simulink model "testMPCWalkingPatternGen"  (R2019b)
settings: Solver=VariableStepAuto  StartTime=0.0  StopTime=10.0  RelTol=1e-3
undefined symbols (not defined in the file or in its folder): numOutputs, predictionHorizon, stepLength, stepTime, stepWidth, Ts, zc
libraries: cstblocks x2, mpclib x2, simulink x1
settings Model: Creator=csantacr  LastModifiedBy=scastro
settings DataIOCC: ReturnWorkspaceOutputs=off
settings DebuggingCC: ArithmeticOperatorsInVariantConditions=warning
settings SFSimCC: CustomCodeUndefinedFunction=UseInterfaceOnly

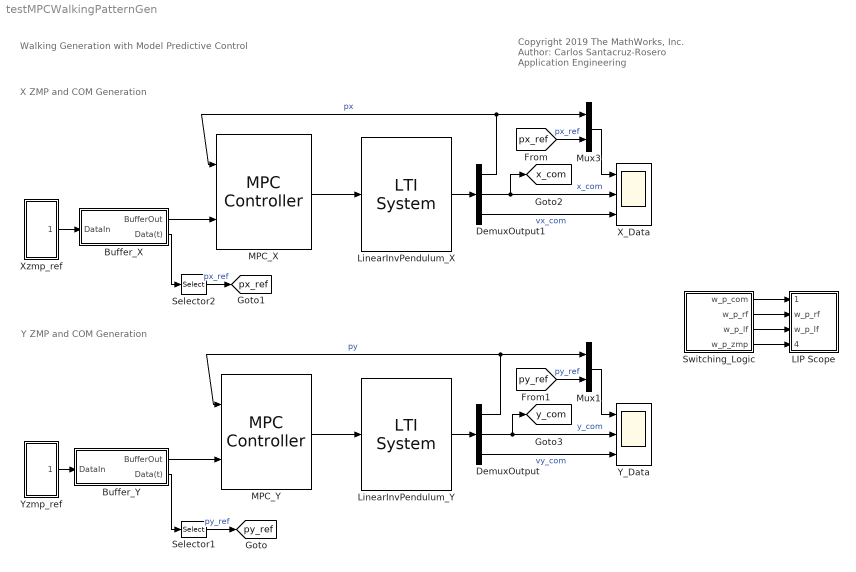
== system testMPCWalkingPatternGen ==
  note: Copyright 2019 The MathWorks, Inc.
      | Author: Carlos Santacruz-Rosero
      | Application Engineering
  note: Walking Generation with Model Predictive Control
  note: Y ZMP and COM Generation
  note: X ZMP and COM Generation
  Buffer_X : Subsystem
  Buffer_Y : Subsystem
  DemuxOutput : Demux  Outputs=3
  DemuxOutput1 : Demux  Outputs=3
  LIP Scope : Subsystem
  LinearInvPendulum_X : cstblocks/LTI System  sys=lip_x_d  IC=[0;0;0]  mask(LTI Block){}
      mask Display:
      | % This is a new mask on top of the base mask.
      | % Use "View base mask" link below to see the base mask.
      | image('lipm.jpg')
  LinearInvPendulum_Y : cstblocks/LTI System  sys=lip_y_d  IC=[0;0;0]  mask(LTI Block){}
      mask Display:
      | % This is a new mask on top of the base mask.
      | % Use "View base mask" link below to see the base mask.
      | image('lipm.jpg');
  MPC_X : mpclib/MPC Controller  SCDEnableBlockLinearizationSpecification=on  mpcobj=mpc1  is_multiple=0  enable_value=0  return_u0=off  updateMPCinCallerWorkspace=on  md_inport=off  mv_inport=off  uref_inport=off  return_cost=off  return_mvseq=off  return_qpstatus=off  return_xseq=off  return_state=off  return_ovseq=off  state_inport=off  umin_inport=off  umax_inport=off  ymin_inport=off  ymax_inport=off  cc_inport=off  ywt_inport=off  uwt_inport=off  duwt_inport=off  rhoeps_inport=off  pm_inport=off  MaximumP=10  HorizonChoice=FixedHorizon  n_ts=0.005  n_p=300  n_mv=1  n_md=0  n_ud=0  n_mo=1  n_uo=2  BlockDataType=double  SampleTimeInherited=off  switch_inport=off
  MPC_Y : mpclib/MPC Controller  SCDEnableBlockLinearizationSpecification=on  mpcobj=mpc1  is_multiple=0  enable_value=0  return_u0=off  updateMPCinCallerWorkspace=on  md_inport=off  mv_inport=off  uref_inport=off  return_cost=off  return_mvseq=off  return_qpstatus=off  return_xseq=off  return_state=off  return_ovseq=off  state_inport=off  umin_inport=off  umax_inport=off  ymin_inport=off  ymax_inport=off  cc_inport=off  ywt_inport=off  uwt_inport=off  duwt_inport=off  rhoeps_inport=off  pm_inport=off  MaximumP=10  HorizonChoice=FixedHorizon  n_ts=0.005  n_p=300  n_mv=1  n_md=0  n_ud=0  n_mo=1  n_uo=2  BlockDataType=double  SampleTimeInherited=off  switch_inport=off
  Mux1 : Mux  Inputs=2
  Mux3 : Mux  Inputs=2
  Selector1 : Selector  InputPortWidth=3  IndexOptions=Index vector (dialog)  Indices=[1]  OutputSizes=1
  Selector2 : Selector  InputPortWidth=3  IndexOptions=Index vector (dialog)  Indices=[1]  OutputSizes=1
  Switching_Logic : Subsystem
  X_Data : Scope  NumInputPorts=3
  Xzmp_ref : Subsystem
  Y_Data : Scope  NumInputPorts=3
  Yzmp_ref : Subsystem
  tag scope: px_ref=global, py_ref=global, x_com=global, y_com=global
  wires:
  LinearInvPendulum_Y/1 -> DemuxOutput/1
  DemuxOutput/1 -> Mux1/1, MPC_Y/1  "py"
  DemuxOutput/2 -> Y_Data/2, [y_com]  "y_com"
  DemuxOutput/3 -> Y_Data/3  "vy_com"
  MPC_Y/1 -> LinearInvPendulum_Y/1
  [py_ref] -> Mux1/2  "py_ref"
  Mux1/1 -> Y_Data/1
  Buffer_Y/2(Data(t)) -> Selector1/1
  Buffer_Y/1(BufferOut) -> MPC_Y/2
  Buffer_X/1(BufferOut) -> MPC_X/2
  Buffer_X/2(Data(t)) -> Selector2/1
  MPC_X/1 -> LinearInvPendulum_X/1
  Mux3/1 -> X_Data/1
  [px_ref] -> Mux3/2  "px_ref"
  DemuxOutput1/3 -> X_Data/3  "vx_com"
  DemuxOutput1/2 -> X_Data/2, [x_com]  "x_com"
  DemuxOutput1/1 -> Mux3/1, MPC_X/1  "px"
  LinearInvPendulum_X/1 -> DemuxOutput1/1
  Xzmp_ref/1(X_ref) -> Buffer_X/1(DataIn)
  Yzmp_ref/1(Y_ref) -> Buffer_Y/1(DataIn)
  Selector2/1 -> [px_ref]  "px_ref"
  Selector1/1 -> [py_ref]  "py_ref"
  Switching_Logic/1(w_p_com) -> LIP Scope/1(w_p_com)
  Switching_Logic/2(w_p_rf) -> LIP Scope/2(w_p_rf)
  Switching_Logic/3(w_p_lf) -> LIP Scope/3(w_p_lf)
  Switching_Logic/4(w_p_zmp) -> LIP Scope/4(w_p_zmp)

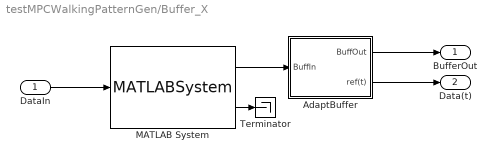
== system testMPCWalkingPatternGen/Buffer_X ==
  DataIn : Inport
  AdaptBuffer : Subsystem
  MATLAB System : MATLABSystem  System=FIFOBuffer  Capacity=predictionHorizon  NumStates=numOutputs  SampleTime=Ts  FillBufferAtStartup=on  BufferStartupFillupData=zeros(numOutputs,predictionHorizon)  SimulateUsing=Code generation
      mask Type: FIFOBuffer
      mask Display:
      | disp('FIFOBuffer');
      | port_label('input',1,'dataIn');
      | port_label('output',1,'buffer');
      | port_label('output',2,'isFull');
  Terminator : Terminator
  BufferOut : Outport
  Data(t) : Outport  Port=2
  wires:
  AdaptBuffer/2(ref(t)) -> Data(t)/1
  DataIn/1 -> MATLAB System/1
  MATLAB System/2 -> Terminator/1
  AdaptBuffer/1(BuffOut) -> BufferOut/1
  MATLAB System/1 -> AdaptBuffer/1(BuffIn)

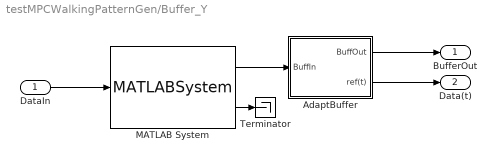
== system testMPCWalkingPatternGen/Buffer_Y ==
  DataIn : Inport
  AdaptBuffer : Subsystem
  MATLAB System : MATLABSystem  System=FIFOBuffer  Capacity=predictionHorizon  NumStates=numOutputs  SampleTime=Ts  FillBufferAtStartup=on  BufferStartupFillupData=zeros(numOutputs,predictionHorizon)  SimulateUsing=Code generation
      mask Type: FIFOBuffer
      mask Display:
      | disp('FIFOBuffer');
      | port_label('input',1,'dataIn');
      | port_label('output',1,'buffer');
      | port_label('output',2,'isFull');
  Terminator : Terminator
  BufferOut : Outport
  Data(t) : Outport  Port=2
  wires:
  MATLAB System/1 -> AdaptBuffer/1(BuffIn)
  AdaptBuffer/1(BuffOut) -> BufferOut/1
  MATLAB System/2 -> Terminator/1
  DataIn/1 -> MATLAB System/1
  AdaptBuffer/2(ref(t)) -> Data(t)/1

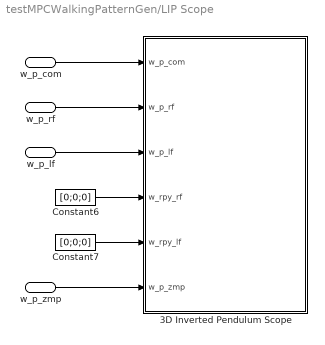
== system testMPCWalkingPatternGen/LIP Scope ==
  w_p_com : Inport
  w_p_rf : Inport  Port=2
  w_p_lf : Inport  Port=3
  w_p_zmp : Inport  Port=4
  3D Inverted Pendulum Scope : Subsystem  TreatAsAtomicUnit=on  mask(3D Inverted Pendulum Scope){x_min=-0.1, x_max=1, y_min=-0.5, y_max=0.5, z_min=0, z_max=0.4, fl=0.1, fw=0.05}
      mask prompts: x_min "X min"; x_max "X max"; y_min "Y min"; z_min "Z min"; z_max "Z max"; fl "Base Length"; fw "Base Width"
      mask help: Plots the 3D Inverted Pendulum. It assumes the pivot is in the middle of the base.
  Constant6 : Constant  Value=[0;0;0]
  Constant7 : Constant  Value=[0;0;0]
  wires:
  Constant6/1 -> 3D Inverted Pendulum Scope/4(w_rpy_rf)
  Constant7/1 -> 3D Inverted Pendulum Scope/5(w_rpy_lf)
  w_p_rf/1 -> 3D Inverted Pendulum Scope/2(w_p_rf)
  w_p_lf/1 -> 3D Inverted Pendulum Scope/3(w_p_lf)
  w_p_com/1 -> 3D Inverted Pendulum Scope/1(w_p_com)
  w_p_zmp/1 -> 3D Inverted Pendulum Scope/6(w_p_zmp)

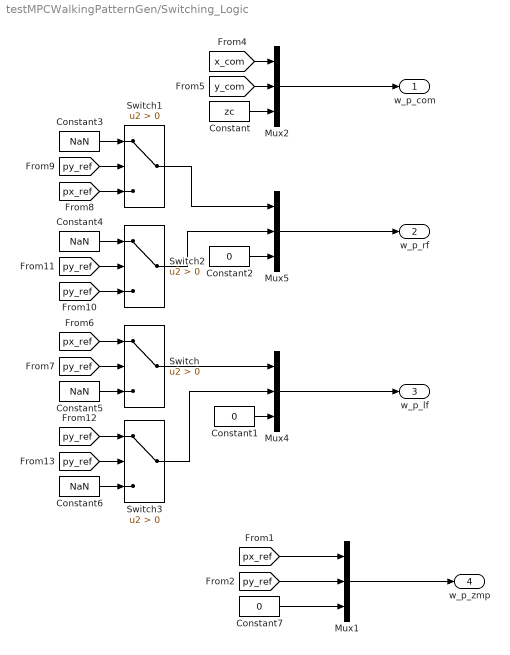
== system testMPCWalkingPatternGen/Switching_Logic ==
  Constant : Constant  Value=zc
  Constant1 : Constant  Value=0
  Constant2 : Constant  Value=0
  Constant{3..6} (4 alike) : Constant  Value=NaN
  Constant7 : Constant  Value=0
  Mux{1..2,4..5} (4 alike) : Mux  Inputs=3
  Switch{,1..3} (4 alike) : Switch  Criteria=u2 > Threshold
  w_p_com : Outport
  w_p_rf : Outport  Port=2
  w_p_lf : Outport  Port=3
  w_p_zmp : Outport  Port=4
  wires:
  Switch/1 -> Mux4/1
  Constant2/1 -> Mux5/3
  Mux5/1 -> w_p_rf/1
  Mux4/1 -> w_p_lf/1
  Constant/1 -> Mux2/3
  Switch1/1 -> Mux5/1
  [px_ref] -> Switch/1
  [py_ref] -> Switch1/2
  Constant6/1 -> Switch3/3
  Constant5/1 -> Switch/3
  [px_ref] -> Switch1/3
  Constant4/1 -> Switch2/1
  Mux2/1 -> w_p_com/1
  [y_com] -> Mux2/2
  [x_com] -> Mux2/1
  Constant3/1 -> Switch1/1
  Switch2/1 -> Mux5/2
  [py_ref] -> Switch2/2
  [py_ref] -> Switch2/3
  [py_ref] -> Switch/2
  Constant1/1 -> Mux4/3
  Switch3/1 -> Mux4/2
  [py_ref] -> Switch3/1
  [py_ref] -> Switch3/2
  Mux1/1 -> w_p_zmp/1
  Constant7/1 -> Mux1/3
  [px_ref] -> Mux1/1
  [py_ref] -> Mux1/2

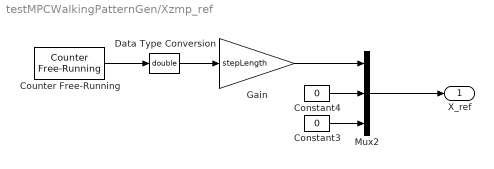
== system testMPCWalkingPatternGen/Xzmp_ref ==
  Constant3 : Constant  Value=0  SampleTime=Ts
  Constant4 : Constant  Value=0  SampleTime=Ts
  Counter Free-Running : simulink/Sources/Counter Free-Running  NumBits=64  tsamp=stepTime
  Data Type Conversion : DataTypeConversion  OutDataTypeStr=double
  Gain : Gain  Gain=stepLength
  Mux2 : Mux  Inputs=3
  X_ref : Outport
  wires:
  Gain/1 -> Mux2/1
  Constant3/1 -> Mux2/3
  Data Type Conversion/1 -> Gain/1
  Counter Free-Running/1 -> Data Type Conversion/1
  Mux2/1 -> X_ref/1
  Constant4/1 -> Mux2/2

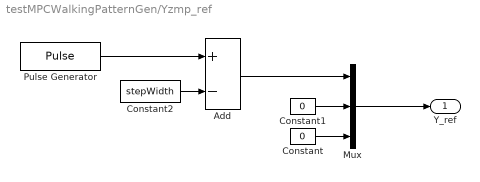
== system testMPCWalkingPatternGen/Yzmp_ref ==
  Add : Sum  Inputs=+-
  Constant : Constant  Value=0  SampleTime=Ts
  Constant1 : Constant  Value=0  SampleTime=Ts
  Constant2 : Constant  Value=stepWidth  SampleTime=Ts
  Mux : Mux  Inputs=3
  Pulse Generator : DiscretePulseGenerator  PulseType=Time based  Amplitude=2*stepWidth  Period=2*stepTime  PulseWidth=50
  Y_ref : Outport
  wires:
  Mux/1 -> Y_ref/1
  Constant1/1 -> Mux/2
  Constant2/1 -> Add/2
  Constant/1 -> Mux/3
  Add/1 -> Mux/1
  Pulse Generator/1 -> Add/1

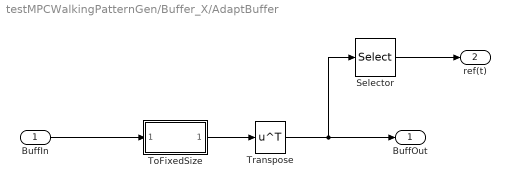
== system testMPCWalkingPatternGen/Buffer_X/AdaptBuffer ==
  BuffIn : Inport
  Selector : Selector  NumberOfDimensions=2  InputPortWidth=3  IndexOptions=Index vector (dialog),Select all  Indices=[1],1  OutputSizes=1,1
  ToFixedSize : MATLAB Function  TreatAsAtomicUnit=on  mask{predictionHorizon=predictionHorizon, numStates=numOutputs}
      mask prompts: predictionHorizon "Prediction Horizon"; numStates "Number of States"
  Transpose : Math  Operator=transpose  SaturateOnIntegerOverflow=on
  BuffOut : Outport
  ref(t) : Outport  Port=2
  wires:
  Selector/1 -> ref(t)/1
  BuffIn/1 -> ToFixedSize/1(buffIn)
  Transpose/1 -> BuffOut/1, Selector/1
  ToFixedSize/1(buffOut) -> Transpose/1

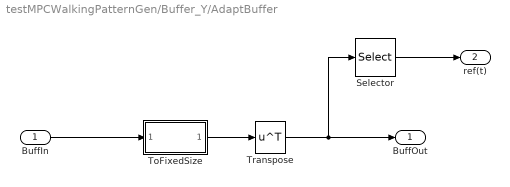
== system testMPCWalkingPatternGen/Buffer_Y/AdaptBuffer ==
  BuffIn : Inport
  Selector : Selector  NumberOfDimensions=2  InputPortWidth=3  IndexOptions=Index vector (dialog),Select all  Indices=[1],1  OutputSizes=1,1
  ToFixedSize : MATLAB Function  TreatAsAtomicUnit=on  mask{predictionHorizon=predictionHorizon, numStates=numOutputs}
      mask prompts: predictionHorizon "Prediction Horizon"; numStates "Number of States"
  Transpose : Math  Operator=transpose  SaturateOnIntegerOverflow=on
  BuffOut : Outport
  ref(t) : Outport  Port=2
  wires:
  ToFixedSize/1(buffOut) -> Transpose/1
  Transpose/1 -> Selector/1, BuffOut/1
  BuffIn/1 -> ToFixedSize/1(buffIn)
  Selector/1 -> ref(t)/1

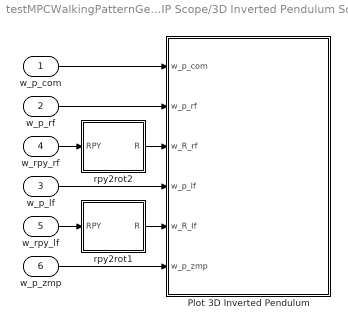
== system testMPCWalkingPatternGen/LIP Scope/3D Inverted Pendulum Scope ==
  w_p_com : Inport
  w_p_rf : Inport  Port=2
  w_p_lf : Inport  Port=3
  w_rpy_rf : Inport  Port=4
  w_rpy_lf : Inport  Port=5
  w_p_zmp : Inport  Port=6
  Plot 3D Inverted Pendulum : MATLAB Function  TreatAsAtomicUnit=on
  rpy2rot1 : Subsystem
  rpy2rot2 : Subsystem
  wires:
  w_rpy_rf/1 -> rpy2rot2/1(RPY)
  w_rpy_lf/1 -> rpy2rot1/1(RPY)
  w_p_lf/1 -> Plot 3D Inverted Pendulum/4(w_p_lf)
  w_p_rf/1 -> Plot 3D Inverted Pendulum/2(w_p_rf)
  w_p_com/1 -> Plot 3D Inverted Pendulum/1(w_p_com)
  rpy2rot2/1(R) -> Plot 3D Inverted Pendulum/3(w_R_rf)
  rpy2rot1/1(R) -> Plot 3D Inverted Pendulum/5(w_R_lf)
  w_p_zmp/1 -> Plot 3D Inverted Pendulum/6(w_p_zmp)

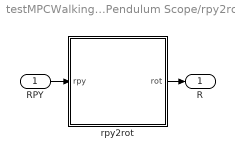
== system testMPCWalkingPatternGen/LIP Scope/3D Inverted Pendulum Scope/rpy2rot1 ==
  RPY : Inport
  rpy2rot : MATLAB Function  TreatAsAtomicUnit=on
  R : Outport
  wires:
  RPY/1 -> rpy2rot/1(rpy)
  rpy2rot/1(rot) -> R/1

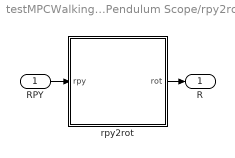
== system testMPCWalkingPatternGen/LIP Scope/3D Inverted Pendulum Scope/rpy2rot2 ==
  RPY : Inport
  rpy2rot : MATLAB Function  TreatAsAtomicUnit=on
  R : Outport
  wires:
  RPY/1 -> rpy2rot/1(rpy)
  rpy2rot/1(rot) -> R/1

== matlab function testMPCWalkingPatternGen/Buffer_X/AdaptBuffer/ToFixedSize ==
  data: buffIn input size=[numStates,predictionHorizon]; buffOut output size=[numStates,predictionHorizon]; predictionHorizon parameter size=1; numStates parameter size=1
function buffOut = fcn(buffIn,predictionHorizon, numStates)

buffOut = buffIn(1:numStates,1:predictionHorizon);

== matlab function testMPCWalkingPatternGen/Buffer_Y/AdaptBuffer/ToFixedSize ==
  data: buffIn input size=[numStates,predictionHorizon]; buffOut output size=[numStates,predictionHorizon]; predictionHorizon parameter size=1; numStates parameter size=1
function buffOut = fcn(buffIn,predictionHorizon, numStates)

buffOut = buffIn(1:numStates,1:predictionHorizon);

== matlab function testMPCWalkingPatternGen/LIP Scope/3D Inverted Pendulum Scope/rpy2rot2/rpy2rot ==
  data: rpy input size=[3]; rot output size=[3 3]
function rot = rpy2rot(rpy)
%#codegen
%%RPY2ROT Transforms from RPY angles to rotation matrix
% rpy is a vector of three RPY angles
% rot is a rotation matrix of 3x3
rot = zeros(3,3);
x = rpy(1);
y = rpy(2);
z = rpy(3);

ca = cos(x); sa = sin(x);
cb = cos(y); sb = sin(y);
cc = cos(z); sc = sin(z);


rot(1,1) = cb*cc;
rot(1,2) = sa*sb*cc - ca*sc;
rot(1,3) = ca*sb*cc + sa*sc;
rot(2,1) = cb*sc;
rot(2,2) = sa*sb*sc + ca*cc;
rot(2,3) = ca*sb*sc - sa*cc;
rot(3,1) = -sb;
rot(3,2) = sa*cb;
rot(3,3) = ca*cb;

== matlab function testMPCWalkingPatternGen/LIP Scope/3D Inverted Pendulum Scope/Plot 3D Inverted Pendulum ==
  data: w_p_com input; w_p_rf input; w_R_rf input; w_p_lf input; w_R_lf input; w_p_zmp input; x_min parameter size=1; x_max parameter size=1; y_min parameter size=1; y_max parameter size=1; z_min parameter size=1; z_max parameter size=1; fl parameter size=1; fw parameter size=1
function drawPendulum(w_p_com, w_p_rf, w_R_rf,  w_p_lf, w_R_lf, w_p_zmp, ... 
                      x_min, x_max, y_min, y_max, z_min, z_max, ...
                      fl, fw)  

persistent init;
persistent hrf;
persistent hlf;
persistent hcom;
persistent hcomTrace;
persistent hzmpTrace;
persistent comBuff;
persistent zmpBuff;
persistent counter;
persistent hsphere;
persistent p;
persistent r_or;
persistent c_or;



%% Initialization code
if isempty(init)
    % Reuse figure if it already exists
    fh = findobj('type','figure','name','Linear Inverted Pendulum');
    if isempty(fh) 
        figureHandle = figure('Name', 'Linear Inverted Pendulum');
    else
        figureHandle = fh;
    end
    figure(figureHandle)
    clf(figureHandle)


    % Clear the figure
    figureAxis = axes(figureHandle);
    cla(figureAxis);
    
    % create right foot vertices
    w_p_rf = [0;0;0];
    rf_fe = w_p_rf + w_R_rf * [ fl/2; -fw/2; 0];
    rf_be = w_p_rf + w_R_rf * [-fl/2; -fw/2; 0];
    rf_fi = w_p_rf + w_R_rf * [ fl/2;  fw/2; 0];
    rf_bi = w_p_rf + w_R_rf *  [-fl/2;  fw/2; 0];
    rf = [rf_fe'; rf_be';  rf_bi'; rf_fi'; rf_fe'];
    % create left foot vertices
    w_p_lf = [0;0;0];
    lf_fe = w_p_lf + w_R_lf * [ fl/2;  fw/2; 0];
    lf_be = w_p_lf + w_R_lf * [-fl/2;  fw/2; 0];
    lf_fi = w_p_lf + w_R_lf * [ fl/2; -fw/2; 0];
    lf_bi = w_p_lf + w_R_lf * [-fl/2; -fw/2; 0];
    lf = [lf_fe'; lf_be';  lf_bi'; lf_fi'; lf_fe'];
    % create CoM vertices
    com = w_p_com';
    % plot right foot
    hrf = plot3(rf(:, 1), rf(:, 2), rf(:, 3),'k','lineWidth', 2.5);
    % plot left foot
    hold on;
    hlf = plot3(lf(:, 1), lf(:, 2), lf(:, 3),'k','lineWidth', 2.5);
    axis([x_min, x_max, y_min, y_max, z_min, z_max]);
%     % plot CoM
%     hcom = plot3(com(:, 1), com(:, 2), com(:, 3), '-g*','lineWidth', 30.5, ...
%         'MarkerSize', 30);
    
    % plot CoM trace. 
    comBuff = nan(3,10000);
    counter = 1;
    comBuff(:,counter) = [com(:, 1); com(:, 2); com(:, 3)];
    hcomTrace = plot3(comBuff(1,:),comBuff(2,:) ,comBuff(3,:), '-b','lineWidth', 1.5);   
    % plot ZMP trace
    zmpBuff = nan(3,10000);
    zmpBuff(:,counter) = [w_p_zmp(1); w_p_zmp(2); w_p_zmp(3)];
    hzmpTrace = plot3(zmpBuff(1,:),zmpBuff(2,:) ,zmpBuff(3,:), '-m','lineWidth', 1.5);     

    
    
    % plot sphere
    radius = 0.1;
    
    %[xe,ye,ze] = sphere(20);
    s = load('sphereData.mat');
    xe = s.xe;
    ye = s.ye;
    ze = s.ze;
    
    xe = radius * xe;
    ye = radius * ye;
    ze = radius * ze;
    
    [r_or,c_or] = size(xe);
    p = [xe(:)';ye(:)';ze(:)';ones(1,numel(xe))];
    
    T = eye(4);
    T(1:3,4) = [com(:, 1); com(:, 2); com(:, 3)];    
    w_p = T * p;
    xe = reshape(w_p(1,:),r_or,c_or); 
    ye = reshape(w_p(2,:),r_or,c_or);
    ze = reshape(w_p(3,:),r_or,c_or);
    hold on;
    hsphere = surf(xe,ye,ze, ...
                    'FaceAlpha', 0.5,...
                    'FaceColor', 'green',...
                    'EdgeAlpha', 0.3,...
                    'EdgeColor', 'black');
    hold off;
    
    grid minor;
    init = 1;
    xlabel('X');ylabel('Y');zlabel('Z');
    title('Generated ZMP & COM with MPC');
end


%% Compute vertices
% right foot
rf_fe = w_p_rf + w_R_rf * [ fl/2; -fw/2; 0];
rf_be = w_p_rf + w_R_rf * [-fl/2; -fw/2; 0];
rf_fi = w_p_rf + w_R_rf * [ fl/2;  fw/2; 0];
rf_bi = w_p_rf + w_R_rf *  [-fl/2;  fw/2; 0];
rf = [rf_fe'; rf_be';  rf_bi'; rf_fi'; rf_fe'];
% left foot
lf_fe = w_p_lf + w_R_lf * [ fl/2;  fw/2; 0];
lf_be = w_p_lf + w_R_lf * [-fl/2;  fw/2; 0];
lf_fi = w_p_lf + w_R_lf * [ fl/2; -fw/2; 0];
lf_bi = w_p_lf + w_R_lf * [-fl/2; -fw/2; 0];
lf = [lf_fe'; lf_be';  lf_bi'; lf_fi'; lf_fe'];
% CoM
com = w_p_com';
% update plot data
set(hrf, 'xdata', rf(:, 1)', 'ydata', rf(:, 2)', 'zdata', rf(:, 3)');
set(hlf, 'xdata', lf(:, 1)', 'ydata', lf(:, 2)', 'zdata', lf(:, 3)');
% set(hcom, 'xdata', com(:, 1)', 'ydata', com(:, 2)', 'zdata', com(:, 3)');

counter = counter + 1;
comBuff(:,counter) = [com(:, 1); com(:, 2); com(:, 3)];
set(hcomTrace, 'xdata', comBuff(1,:), 'ydata', comBuff(2,:), 'zdata', comBuff(3,:));

zmpBuff(:,counter) = [w_p_zmp(1); w_p_zmp(2); w_p_zmp(3)];
set(hzmpTrace, 'xdata', zmpBuff(1,:), 'ydata', zmpBuff(2,:), 'zdata', zmpBuff(3,:));


T = eye(4);
T(1:3,4) = [com(:, 1); com(:, 2); com(:, 3)];    
w_p = T * p;
xe = reshape(w_p(1,:),r_or,c_or); 
ye = reshape(w_p(2,:),r_or,c_or);
ze = reshape(w_p(3,:),r_or,c_or);
set(hsphere, 'xdata', xe, 'ydata', ye, 'zdata', ze);

== matlab function testMPCWalkingPatternGen/LIP Scope/3D Inverted Pendulum Scope/rpy2rot1/rpy2rot ==
  data: rpy input size=[3]; rot output size=[3 3]
function rot = rpy2rot(rpy)
%#codegen
%%RPY2ROT Transforms from RPY angles to rotation matrix
% rpy is a vector of three RPY angles
% rot is a rotation matrix of 3x3
rot = zeros(3,3);
x = rpy(1);
y = rpy(2);
z = rpy(3);

ca = cos(x); sa = sin(x);
cb = cos(y); sb = sin(y);
cc = cos(z); sc = sin(z);


rot(1,1) = cb*cc;
rot(1,2) = sa*sb*cc - ca*sc;
rot(1,3) = ca*sb*cc + sa*sc;
rot(2,1) = cb*sc;
rot(2,2) = sa*sb*sc + ca*cc;
rot(2,3) = ca*sb*sc - sa*cc;
rot(3,1) = -sb;
rot(3,2) = sa*cb;
rot(3,3) = ca*cb;
